simulink model "Ref_RAM"  (R2015b)
settings: Solver=FixedStepDiscrete  SolverMode=SingleTasking  StartTime=0.0  StopTime=SimEnd+Ts2*NTaps*2  RelTol=1e-3
PreLoadFcn:
  | Param_fir
undefined symbols (not defined in the file): NTaps
settings Model: Creator=bogilvie  LastModifiedBy=amatsumo
settings DataIOCC: SaveFormat=Array  SignalLoggingSaveFormat=ModelDataLogs  SaveOutput=off  SignalLogging=off  SaveTime=off
settings OptimizationCC: BlockReduction=off  ConditionallyExecuteInputs=off  DefaultParameterBehavior=Inlined  ExpressionDepthLimit=2147483647  InitFltsAndDblsToZero=on
settings DebuggingCC: AlgebraicLoopMsg=error  UnderspecifiedInitializationDetection=Classic  MergeDetectMultiDrivingBlocksExec=none  SignalResolutionControl=TryResolveAllWithWarning  SolverPrmCheckMsg=warning  SingleTaskRateTransMsg=error  IntegerOverflowMsg=none  ParameterOverflowMsg=warning  ParameterPrecisionLossMsg=none  FcnCallInpInsideContextMsg=UseLocalSettings  StateNameClashWarn=warning  IntegerSaturationMsg=none
settings HardwareCC: ProdBitPerPointer=32  ProdLargestAtomicFloat=None  ProdIntDivRoundTo=Undefined  ProdEndianess=Unspecified  ProdWordSize=32  ProdHWDeviceType=ASIC/FPGA->ASIC/FPGA  ProdEqTarget=off
settings SFSimCC: SFSimEcho=off
settings GRTTargetCC: GeneratePreprocessorConditionals=Disable all  CombineOutputUpdateFcns=off  GRTInterface=on
settings ConfigComp: CovModelRefEnable=Off  CovSFcnEnable=off

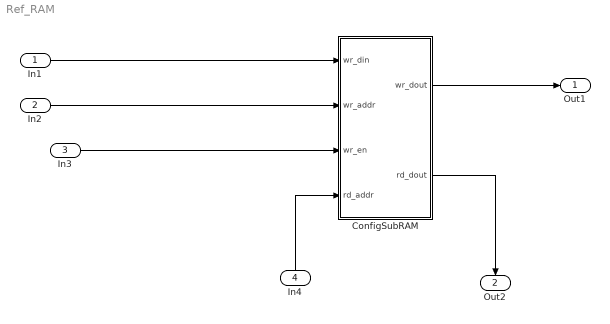
== system Ref_RAM ==
  In1 : Inport  OutDataTypeStr=fixdt('sfix16_En15')  PortDimensions=1  SampleTime=[7.8125000000000002e-05,0]
  In2 : Inport  Port=2  OutDataTypeStr=fixdt('ufix7')  PortDimensions=1  SampleTime=[7.8125000000000002e-05,0]
  In3 : Inport  Port=3  OutDataTypeStr=boolean  PortDimensions=1  SampleTime=[7.8125000000000002e-05,0]
  In4 : Inport  Port=4  OutDataTypeStr=fixdt('ufix7')  PortDimensions=1  SampleTime=[7.8125000000000002e-05,0]
  ConfigSubRAM : Subsystem  mask(Dual-port RAM){ram_size=ceil(log2(NTaps))}
      mask prompts: ram_size "Address port width (2 to 16)"
      mask help:
      | This block simulates a dual-port RAM with two data output ports.
      |
      | The read and write address port width is limited to between 2 to 16 bits.
      mask init:
      | hdlblkmask_dpram;
      settings: ErrorFcn=hdlblkmask_errfcn
      mask Help: helpview([docroot '/toolbox/hdlcoder/ug/hdlcoder_ug.map'],'HDL_dual_port_RAM');
  Out1 : Outport  OutDataTypeStr=fixdt('sfix16_En15')  PortDimensions=1  SampleTime=[7.8125000000000002e-05,0]
  Out2 : Outport  Port=2  OutDataTypeStr=fixdt('sfix16_En15')  PortDimensions=1  SampleTime=[7.8125000000000002e-05,0]
  wires:
  In3/1 -> ConfigSubRAM/3(wr_en)
  In4/1 -> ConfigSubRAM/4(rd_addr)
  In2/1 -> ConfigSubRAM/2(wr_addr)
  In1/1 -> ConfigSubRAM/1(wr_din)
  ConfigSubRAM/1(wr_dout) -> Out1/1
  ConfigSubRAM/2(rd_dout) -> Out2/1

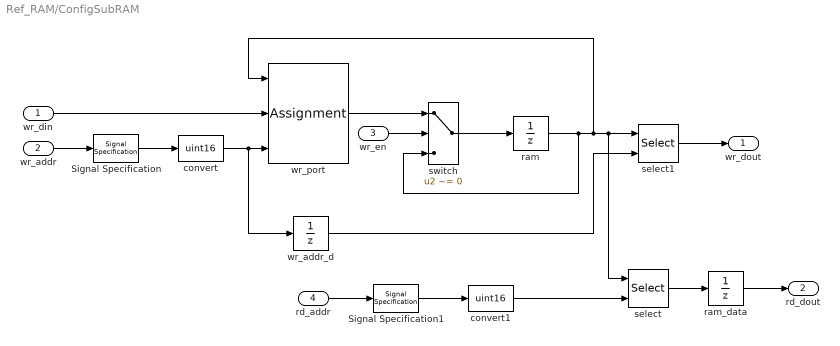
== system Ref_RAM/ConfigSubRAM ==
  wr_din : Inport
  wr_addr : Inport  Port=2
  wr_en : Inport  Port=3  OutDataTypeStr=boolean
  rd_addr : Inport  Port=4
  Signal Specification : SignalSpecification  OutDataTypeStr=fixdt(0,ram_size,0)  Dimensions=1
  Signal Specification1 : SignalSpecification  OutDataTypeStr=fixdt(0,ram_size,0)  Dimensions=1
  convert : DataTypeConversion  OutDataTypeStr=uint16
  convert1 : DataTypeConversion  OutDataTypeStr=uint16
  ram : UnitDelay  SampleTime=-1
  ram_data : UnitDelay  SampleTime=-1
  select : Selector  IndexMode=Zero-based  InputPortWidth=2^ram_size  IndexOptions=Index vector (port)  Indices=[1 3]  OutputSizes=1
  select1 : Selector  IndexMode=Zero-based  InputPortWidth=2^ram_size  IndexOptions=Index vector (port)  Indices=[1 3]  OutputSizes=1
  switch : Switch  Criteria=u2 ~= 0
  wr_addr_d : UnitDelay  SampleTime=-1
  wr_port : Assignment  IndexMode=Zero-based  IndexOptions=Index vector (port)  Indices=1  OutputSizes=[1 1]
  wr_dout : Outport
  rd_dout : Outport  Port=2
  wires:
  ram_data/1 -> rd_dout/1
  Signal Specification/1 -> convert/1
  wr_addr/1 -> Signal Specification/1
  wr_port/1 -> switch/1
  switch/1 -> ram/1
  ram/1 -> wr_port/1, select/1, select1/1, switch/3
  wr_din/1 -> wr_port/2
  wr_en/1 -> switch/2
  rd_addr/1 -> Signal Specification1/1
  select/1 -> ram_data/1
  convert/1 -> wr_port/3, wr_addr_d/1
  convert1/1 -> select/2
  select1/1 -> wr_dout/1
  wr_addr_d/1 -> select1/2
  Signal Specification1/1 -> convert1/1
